simulink model "DemoMPEG"  (Simulink 7.7)
settings: Solver=ode45  StartTime=0.0  StopTime=10  RelTol=1e-3
PreLoadFcn:
  | EbNo = 16; Errors = 188; Bits = 1e8; M = 256; N = 64; Ts = (1/22050); constellation; InnerInterleaverBitTable
undefined symbols (not defined in the file or in its folder): gray, rsgenpoly
libraries: dspmtrx3 x33, simulink x18, commutil2 x6, commblkintrlv2 x4, commblkcod2 x2, vipsnks x2, dspindex x2, commseqgen2 x2, commrandsrc2 x2, commcnvintrlv2 x2, commsink2 x2, commcnvcod2 x2
settings Model: Creator=katsikas  LastModifiedBy=katsikas
settings SimEventsCC: propDiagAttribOutput=1  propDiagFcnCallOutput=1  propDiagStatOutput=0

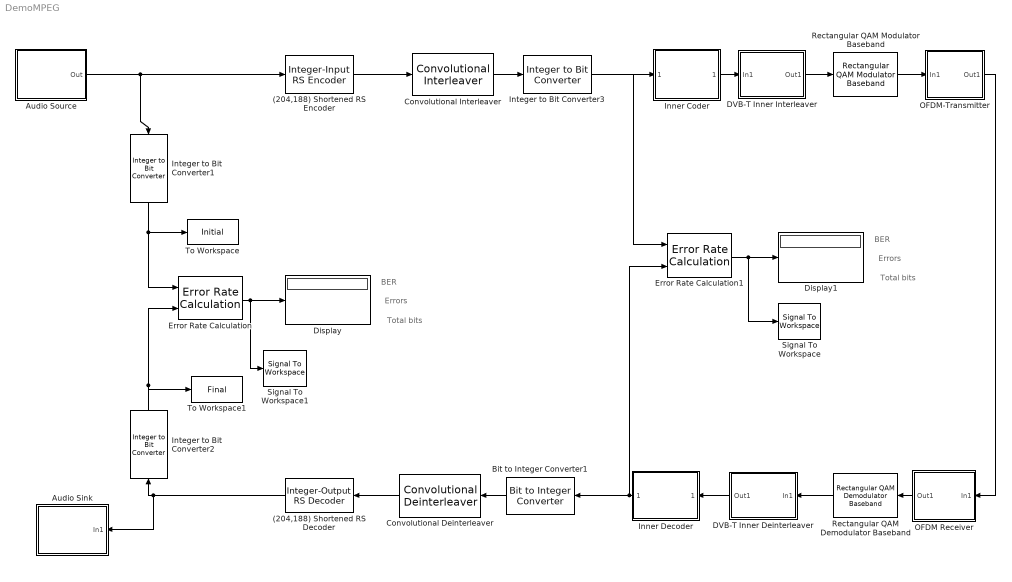
== system DemoMPEG ==
  note: BER
  note: Total bits
  note: Errors
  note: BER
  note: Total bits
  note: Errors
  (204,188) Shortened RS Decoder : commblkcod2/Integer-Output RS Decoder  n=204  k=188  specPrimPoly=off  prPoly=[1 0 1 1]  specGenPoly=off  genPoly=rsgenpoly(7,3)  specPuncture=off  punctVec=[ones(2,1); zeros(2,1)]  specErasurePort=off  showNumErr=off
  (204,188) Shortened RS Encoder : commblkcod2/Integer-Input RS Encoder  n=204  k=188  specPrimPoly=off  prPoly=[1 0 1 1]  specGenPoly=off  genPoly=rsgenpoly(7,3)  specPuncture=off  punctVec=[ones(2,1); zeros(2,1)]
  Audio Sink : Subsystem
  Audio Source : Subsystem
  Bit to Integer Converter1 : commutil2/Bit to Integer Converter  nbits=log2(M)  bitOrder=MSB first  signedOutputValues=Unsigned  outDtype=uint8  outDtypeSigned=Inherit via internal rule
  Convolutional Deinterleaver : commcnvintrlv2/Convolutional Deinterleaver  SystemSampleTime=-1  N=12  B=17  ic=0
  Convolutional Interleaver : commcnvintrlv2/Convolutional Interleaver  SystemSampleTime=-1  N=12  B=17  ic=0
  DVB-T Inner Deinterleaver : Subsystem  mask(DVB-T Inner Deinterleaver){}
      mask init:
      | fullILVec = [(1:126) ...
      |  (rem([0:125]+63,126) +1 + 126     ) ...
      |  (rem([0:125]+105,126)+1 + (2*126) ) ...
      |  (rem([0:125]+42,126) +1 + (3*126) ) ...
      |  (rem([0:125]+21,126) +1 + (4*126) ) ...
      |  (rem([0:125]+84,126) +1 + (5*126) )];
      mask Display: disp('DVB-T\nInner\nDeinterleaver')
  DVB-T Inner Interleaver : Subsystem  mask(DVB-T Inner Interleaver){}
      mask init: same as DemoMPEG/DVB-T Inner Deinterleaver
      mask Display: disp('DVB-T\nInner\nInterleaver')
  Display : Display
  Display1 : Display
  Error Rate Calculation : commsink2/Error Rate Calculation  N=188*17*8  st_delay=0  cp_mode=Entire frame  subframe=[]  PMode=Port  WsName=ErrorVec  RsMode2=off  stop=off  numErr=Errors  maxBits=Bits
  Error Rate Calculation1 : commsink2/Error Rate Calculation  N=1632*6  st_delay=0  cp_mode=Entire frame  subframe=[]  PMode=Port  WsName=ErrorVec  RsMode2=off  stop=off  numErr=100  maxBits=1e8
  Inner Coder : Subsystem
      mask Display: disp('Rate 3/4\nPunctured\nConvolutional\nCode');
  Inner Decoder : Subsystem
      mask Display: disp('Viterbi\nDecoder')
  Integer to Bit Converter1 : commutil2/Integer to Bit Converter  nbits=8  signedInputValues=Unsigned  bitOrder=MSB first  outDtype=boolean
  Integer to Bit Converter2 : commutil2/Integer to Bit Converter  nbits=8  signedInputValues=Unsigned  bitOrder=MSB first  outDtype=boolean
  Integer to Bit Converter3 : commutil2/Integer to Bit Converter  nbits=log2(M)  signedInputValues=Unsigned  bitOrder=MSB first  outDtype=boolean
  OFDM Receiver : Subsystem
  OFDM-Transmitter : Subsystem
  Rectangular QAM Demodulator Baseband : commdigbbndam3/Rectangular QAM Demodulator Baseband  M=N  PowType=Average Power  MinDist=2  AvgPow=1  PeakPow=1  Ph=0  Dec=User-defined  Mapping=map_constellation  OutType=Bit  DecType=Hard decision  VarSource=Dialog  Variance=1  outDtype1=boolean  outDtype2=Inherit via internal rule  derotateFactorWordLen=16  denormFactorWordLen=16  prodOutWordLen=32  prodOutRoundingMode=Floor  prodOutOverflowMode=Wrap  sumWordLen=32
  Rectangular QAM Modulator Baseband : commdigbbndam3/Rectangular QAM Modulator Baseband  M=N  InType=Bit  Enc=User-defined  Mapping=map_constellation  PowType=Average Power  MinDist=2  AvgPow=1  PeakPow=1  Ph=0  outDtype=double  outWordLen=16  outUDDataType=sfix(16)  outFracLenMode=Best precision  outFracLen=15
  Signal To Workspace : SignalToWorkspace  VariableName=BER1  SaveFormat=Array  Save2DMode=2-D array (concatenate along first dimension)
      settings: CopyFcn=dspblkcopystw(gcbh);
  Signal To Workspace1 : SignalToWorkspace  VariableName=BER  SaveFormat=Array  Save2DMode=2-D array (concatenate along first dimension)
      settings: CopyFcn=dspblkcopystw(gcbh);  MaxDataPoints=1
  To Workspace : ToWorkspace  VariableName=Initial  SampleTime=-1  SaveFormat=Array
  To Workspace1 : ToWorkspace  VariableName=Final  SampleTime=-1  SaveFormat=Array
  wires:
  Error Rate Calculation/1 -> Display/1, Signal To Workspace1/1
  Integer to Bit Converter2/1 -> Error Rate Calculation/2, To Workspace1/1
  (204,188) Shortened RS Decoder/1 -> Integer to Bit Converter2/1, Audio Sink/1(In1)
  Rectangular QAM Modulator Baseband/1 -> OFDM-Transmitter/1(In1)
  Convolutional Interleaver/1 -> Integer to Bit Converter3/1
  Convolutional Deinterleaver/1 -> (204,188) Shortened RS Decoder/1
  (204,188) Shortened RS Encoder/1 -> Convolutional Interleaver/1
  Error Rate Calculation1/1 -> Display1/1, Signal To Workspace/1
  Integer to Bit Converter3/1 -> Inner Coder/1(Uncoded symbols), Error Rate Calculation1/1
  Rectangular QAM Demodulator Baseband/1 -> DVB-T Inner Deinterleaver/1(In1)
  Bit to Integer Converter1/1 -> Convolutional Deinterleaver/1
  Inner Coder/1(Coded bits) -> DVB-T Inner Interleaver/1(In1)
  Inner Decoder/1(Decoded symbols) -> Bit to Integer Converter1/1, Error Rate Calculation1/2
  DVB-T Inner Interleaver/1(Out1) -> Rectangular QAM Modulator Baseband/1
  DVB-T Inner Deinterleaver/1(Out1) -> Inner Decoder/1(Received bits)
  OFDM Receiver/1(Out1) -> Rectangular QAM Demodulator Baseband/1
  OFDM-Transmitter/1(Out1) -> OFDM Receiver/1(In1)
  Integer to Bit Converter1/1 -> Error Rate Calculation/1, To Workspace/1
  Audio Source/1(Out) -> Integer to Bit Converter1/1, (204,188) Shortened RS Encoder/1

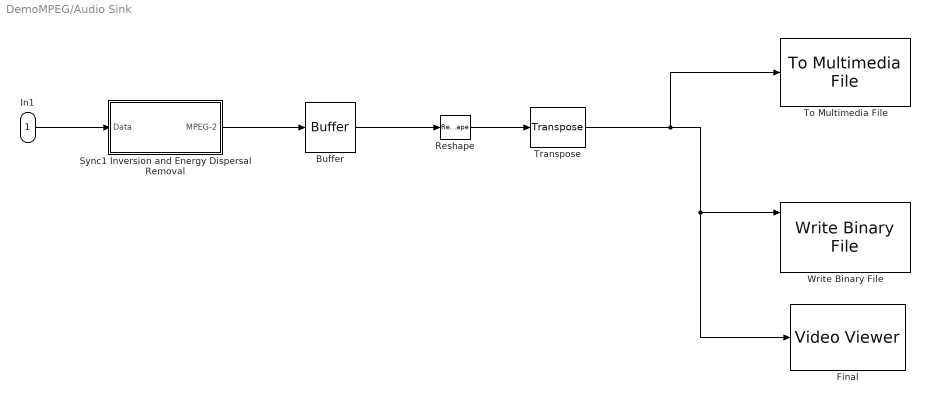
== system DemoMPEG/Audio Sink ==
  In1 : Inport
  Buffer : Buffer  N=120*160  TreatMby1Signals=One channel
  Final : vipsnks/Video Viewer  inputType=Obsolete7b  imagePorts=One multidimensional signal  useColorMap=off  colormapValue=gray(256)  specRange=off  minInputVal=0  maxInputVal=255  FigPos=[730 1122 458 411]  AxisZoom=on  trueSizedOnce=on  OpenAtMdlStart=on
  Reshape : Reshape  OutputDimensionality=Customize  OutputDimensions=[160,120]
  Sync1 Inversion and Energy Dispersal Removal : Subsystem
  To Multimedia File : dspsnks4/To Multimedia File  outputFilename=output.avi  streamSelection=Video only  videoCompressor=None (uncompressed)  audioCompressor=None (uncompressed)  imagePorts=One multidimensional signal  fileType=AVI  audioDatatype=Determine from input data type  fourcc=RGB
  Transpose : dspmtrx3/Transpose  SystemSampleTime=-1  Hermitian=off  overflowFlag=off
  Write Binary File : vipsnks/Write Binary File  FileName=output.bin  VideoFormat=Four character codes  FOURCC=I420  BitStreamFormat=Planar  NumInputs=3  ComponentOrder=[1 2 3]  Interlaced=off  LineOrdering=Top line first  InheritBits=on  Component1=Y'  Component2=Cb  Component3=Cr  Component4=Alpha  Bits1=8  Bits2=8  Bits3=8  Bits4=0  SignedInput=off  FileEndian=Little endian
  wires:
  Reshape/1 -> Transpose/1
  Buffer/1 -> Reshape/1
  In1/1 -> Sync1 Inversion and Energy Dispersal Removal/1(Data)
  Transpose/1 -> Final/1, Write Binary File/1, To Multimedia File/1
  Sync1 Inversion and Energy Dispersal Removal/1(MPEG-2) -> Buffer/1

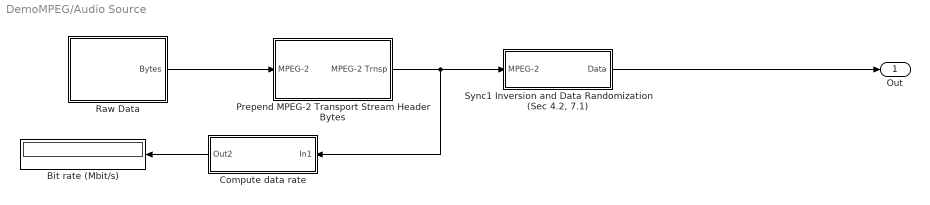
== system DemoMPEG/Audio Source ==
  Bit rate (Mbit/s) : Display
      settings: Format=bank
  Compute data rate : Subsystem
      mask Display: disp(sprintf('Compute Bit\nRate (Mbit/s)'))
  Prepend MPEG-2 Transport Stream Header Bytes : Subsystem
      mask Display: disp(sprintf('Prepend MPEG-2\nTransportStream\nHeader Bytes'))
  "Raw Data " : Subsystem
  "Sync1 Inversion and Data Randomization (Sec 4.2, 7.1)" : Subsystem
  Out : Outport
  wires:
  Prepend MPEG-2 Transport Stream Header Bytes/1(MPEG-2 Trnsp) -> "Sync1 Inversion and Data Randomization (Sec 4.2, 7.1)"/1(MPEG-2), Compute data rate/1(In1)
  "Sync1 Inversion and Data Randomization (Sec 4.2, 7.1)"/1(Data) -> Out/1
  "Raw Data "/1(Bytes) -> Prepend MPEG-2 Transport Stream Header Bytes/1(MPEG-2)
  Compute data rate/1(Out2) -> Bit rate (Mbit/s)/1

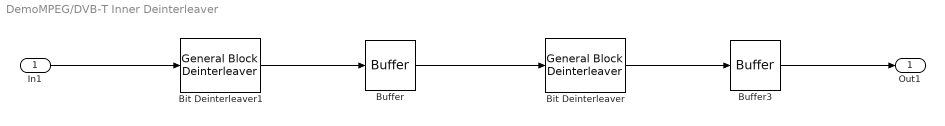
== system DemoMPEG/DVB-T Inner Deinterleaver ==
  In1 : Inport
  Bit Deinterleaver : commblkintrlv2/General Block Deinterleaver  elements=BitInterleaverTable
  Bit Deinterleaver1 : commblkintrlv2/General Block Deinterleaver  elements=SymbolInterleaverTable
  Buffer : Buffer  N=756  TreatMby1Signals=One channel
  Buffer3 : Buffer  N=2176  TreatMby1Signals=One channel
  Out1 : Outport
  wires:
  In1/1 -> Bit Deinterleaver1/1
  Buffer3/1 -> Out1/1
  Buffer/1 -> Bit Deinterleaver/1
  Bit Deinterleaver/1 -> Buffer3/1
  Bit Deinterleaver1/1 -> Buffer/1

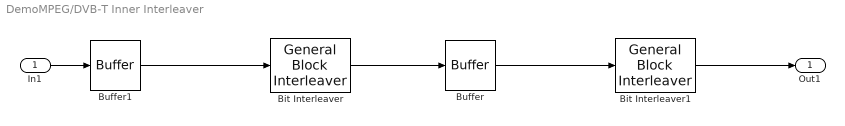
== system DemoMPEG/DVB-T Inner Interleaver ==
  In1 : Inport
  Bit Interleaver : commblkintrlv2/General Block Interleaver  elements=BitInterleaverTable
  Bit Interleaver1 : commblkintrlv2/General Block Interleaver  elements=SymbolInterleaverTable
  Buffer : Buffer  N=9072  TreatMby1Signals=One channel
  Buffer1 : Buffer  N=756  TreatMby1Signals=One channel
  Out1 : Outport
  wires:
  In1/1 -> Buffer1/1
  Buffer/1 -> Bit Interleaver1/1
  Buffer1/1 -> Bit Interleaver/1
  Bit Interleaver/1 -> Buffer/1
  Bit Interleaver1/1 -> Out1/1

== system DemoMPEG/Inner Coder ==
  Uncoded symbols : Inport
  Convolutional  Encoder : commcnvcod2/Convolutional Encoder  trellis=poly2trellis(7, [171 133])  opMode=Continuous  DelayedResetAction=off  hasIniStPort=off  hasFinStPort=off  usePuncVector=on  punctureVector=[1 1 0 1 1 0]'  reset=Unused parameter value
  Coded bits : Outport
  wires:
  Convolutional  Encoder/1 -> Coded bits/1
  Uncoded symbols/1 -> Convolutional  Encoder/1

== system DemoMPEG/Inner Decoder ==
  note: Align on 1632-bit
      | frame boundary
  Received bits : Inport
  Delay : dspsigops/Delay  InputProcessing=Columns as channels (frame based)  dly_unit=Samples  delay=584+69  ic_detail=off  dif_ic_for_ch=off  dif_ic_for_dly=off  ic=0  reset_popup=None
  Viterbi Decoder : commcnvcod2/Viterbi Decoder  trellis=poly2trellis(7, [171 133])  isPunctured=on  punctureVector=[1 1 0 1 1 0]'  erasures=off  dectype=Hard decision  runSigValErrCheck=off  nsdecb=4  smWordLength=16  tbdepth=136  opmode=Continuous  reset=off  outDataType=boolean
  Decoded symbols : Outport
  wires:
  Viterbi Decoder/1 -> Delay/1
  Received bits/1 -> Viterbi Decoder/1
  Delay/1 -> Decoded symbols/1

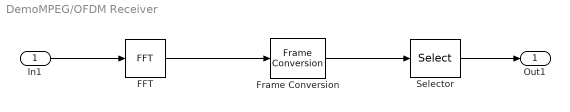
== system DemoMPEG/OFDM Receiver ==
  In1 : Inport
  FFT : dspxfrm3/FFT  CompMethod=Table lookup  TableOpt=NEW  TableOptActive=Speed  BitRevOrder=off  InheritFFTLength=on  FFTLength=64  RowConvenienceOn=on  SkipNorm=off  firstCoeffDataTypeStr=Inherit: Same word length as input  firstCoeffLastDataTypeStr=Inherit: Same word length as input  outputMin=[]  outputMax=[]  roundingMode=Floor  overflowMode=off
  Frame Conversion : FrameConversion
  Selector : Selector  NumberOfDimensions=2  InputPortWidth=3  IndexOptions=Index vector (dialog),Select all  Indices=[1:756 1293:2048],1  OutputSizes=1,1
  Out1 : Outport
  wires:
  FFT/1 -> Frame Conversion/1
  Frame Conversion/1 -> Selector/1
  In1/1 -> FFT/1
  Selector/1 -> Out1/1

== system DemoMPEG/OFDM-Transmitter ==
  In1 : Inport
  IFFT : dspxfrm3/IFFT  CompMethod=Table lookup  TableOpt=NEW  TableOptActive=Speed  BitRevOrder=off  cs_in=off  SkipNorm=on  InheritFFTLength=on  FFTLength=64  mode=Complex  outSamplingMode=Frame based  RowConvenienceOn=on  firstCoeffDataTypeStr=Inherit: Same word length as input  firstCoeffLastDataTypeStr=Inherit: Same word length as input  outputMin=[]  outputMax=[]  roundingMode=Floor  overflowMode=off
  Pad : dspsigops/Pad  padAlong=Columns  dimsToPad=1  valSrc=Specify via dialog  padVal=0  spec=Output size  padNumOutRowsSpecMethod=User-specified  numOutRows=2048  padNumOutColsSpecMethod=User-specified  numOutCols=1  isVarDimsMode=off  padBeginning=0  padEnd=0  outSizeMode=User-specified  outSize=1  padSigAt=End  trunc_flag=None  roundingMode=Floor  overflowMode=off  truncOrWrapMode=Truncate  wrap_flag=None
  Selector : Selector  NumberOfDimensions=2  InputPortWidth=3  IndexOptions=Index vector (dialog),Select all  Indices=[1:756 1513:2048 757:1512],1  OutputSizes=1,1
  Out1 : Outport
  wires:
  Pad/1 -> Selector/1
  Selector/1 -> IFFT/1
  IFFT/1 -> Out1/1
  In1/1 -> Pad/1

== system DemoMPEG/Audio Sink/Sync1 Inversion and Energy Dispersal Removal ==
  Data : Inport
  Buffer to Superframes : Buffer  N=1504  TreatMby1Signals=One channel
  Rebuffer to Packets : Buffer  N=188  TreatMby1Signals=One channel
  Scrambler-Descrambler : Subsystem
  MPEG-2 : Outport
  wires:
  Data/1 -> Buffer to Superframes/1
  Rebuffer to Packets/1 -> MPEG-2/1
  Buffer to Superframes/1 -> Scrambler-Descrambler/1(Data_In)
  Scrambler-Descrambler/1(Data_Out) -> Rebuffer to Packets/1

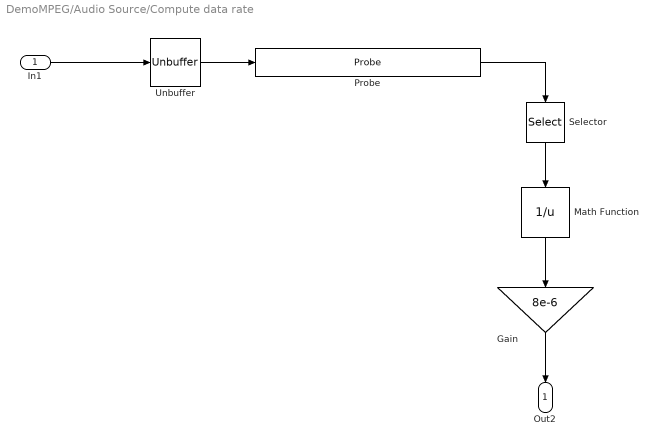
== system DemoMPEG/Audio Source/Compute data rate ==
  In1 : Inport
  Gain : Gain  Gain=8e-6
  Math Function : Math  Operator=reciprocal  SaturateOnIntegerOverflow=on
  Probe : Probe  ProbeWidth=off  ProbeComplexSignal=off
  Selector : Selector  InputPortWidth=2  IndexOptions=Index vector (dialog)  Indices=1  OutputSizes=1
  Unbuffer : Unbuffer  SampleBasedProcessing=Same as frame based
  Out2 : Outport
  wires:
  Probe/1 -> Selector/1
  In1/1 -> Unbuffer/1
  Selector/1 -> Math Function/1
  Math Function/1 -> Gain/1
  Gain/1 -> Out2/1
  Unbuffer/1 -> Probe/1

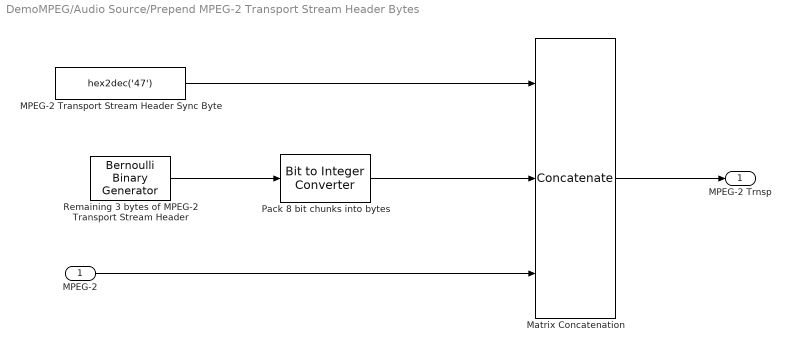
== system DemoMPEG/Audio Source/Prepend MPEG-2 Transport Stream Header Bytes ==
  MPEG-2 : Inport
  MPEG-2 Transport Stream Header Sync Byte : Constant  Value=hex2dec('47')  VectorParams1D=off  OutDataTypeStr=uint8  FramePeriod=(8*188)/9.6e6
      settings: SamplingMode=Frame based
  Matrix Concatenation : Concatenate  NumInputs=3  Mode=Multidimensional array
  Pack 8 bit chunks into bytes : commutil2/Bit to Integer Converter  nbits=8  bitOrder=MSB first  signedOutputValues=Unsigned  outDtype=uint8  outDtypeSigned=Inherit via internal rule
  Remaining 3 bytes of MPEG-2 Transport Stream Header : commrandsrc2/Bernoulli Binary Generator  SystemSampleTime=-1  P=0.5  seed=61  Ts=(8*188/9.6e6) / (3*8)  frameBased=on  sampPerFrame=3*8  orient=off  outDataType=uint8
  MPEG-2 Trnsp : Outport
  wires:
  MPEG-2 Transport Stream Header Sync Byte/1 -> Matrix Concatenation/1
  Remaining 3 bytes of MPEG-2 Transport Stream Header/1 -> Pack 8 bit chunks into bytes/1
  Matrix Concatenation/1 -> MPEG-2 Trnsp/1
  Pack 8 bit chunks into bytes/1 -> Matrix Concatenation/2
  MPEG-2/1 -> Matrix Concatenation/3

== system DemoMPEG/Audio Source/Raw Data  ==
  184 bytes of MPEG-2 or auxiliary data : commrandsrc2/Bernoulli Binary Generator  SystemSampleTime=-1  P=0.5  seed=61  Ts=(8*188/9.6e6) / (8 * 184)  frameBased=on  sampPerFrame=8 * 184  orient=off  outDataType=uint8
  Pack 8 bit chunks into bytes : commutil2/Bit to Integer Converter  nbits=8  bitOrder=MSB first  signedOutputValues=Unsigned  outDtype=uint8  outDtypeSigned=Inherit via internal rule
  Bytes : Outport
  wires:
  184 bytes of MPEG-2 or auxiliary data/1 -> Pack 8 bit chunks into bytes/1
  Pack 8 bit chunks into bytes/1 -> Bytes/1

== system DemoMPEG/Audio Source/Sync1 Inversion and Data Randomization (Sec 4.2, 7.1) ==
  MPEG-2 : Inport
  Buffer to Superframes : Buffer  N=1504  TreatMby1Signals=One channel
  Rebuffer to Packets : Buffer  N=188  TreatMby1Signals=One channel
  Scrambler-Descrambler : Subsystem
  Data : Outport
  wires:
  MPEG-2/1 -> Buffer to Superframes/1
  Rebuffer to Packets/1 -> Data/1
  Scrambler-Descrambler/1(Data_Out) -> Rebuffer to Packets/1
  Buffer to Superframes/1 -> Scrambler-Descrambler/1(Data_In)

== system DemoMPEG/Audio Sink/Sync1 Inversion and Energy Dispersal Removal/Scrambler-Descrambler ==
  Data_In : Inport
  PRBS : Subsystem
  XOR and Concatenate : Subsystem
  Data_Out : Outport
  wires:
  PRBS/1(PRBS1) -> XOR and Concatenate/2(PRBS1)
  PRBS/2(PRBS2) -> XOR and Concatenate/3(PRBS2)
  PRBS/3(PRBS3) -> XOR and Concatenate/4(PRBS3)
  PRBS/4(PRBS4) -> XOR and Concatenate/5(PRBS4)
  PRBS/5(PRBS5) -> XOR and Concatenate/6(PRBS5)
  PRBS/6(PRBS6) -> XOR and Concatenate/7(PRBS6)
  PRBS/7(PRBS7) -> XOR and Concatenate/8(PRBS7)
  PRBS/8(PRBS8) -> XOR and Concatenate/9(PRBS8)
  Data_In/1 -> XOR and Concatenate/1(Data)
  XOR and Concatenate/1(Out1) -> Data_Out/1

== system DemoMPEG/Audio Source/Sync1 Inversion and Data Randomization (Sec 4.2, 7.1)/Scrambler-Descrambler ==
  Data_In : Inport
  PRBS : Subsystem
  XOR and Concatenate : Subsystem
  Data_Out : Outport
  wires:
  PRBS/1(PRBS1) -> XOR and Concatenate/2(PRBS1)
  PRBS/2(PRBS2) -> XOR and Concatenate/3(PRBS2)
  PRBS/3(PRBS3) -> XOR and Concatenate/4(PRBS3)
  PRBS/4(PRBS4) -> XOR and Concatenate/5(PRBS4)
  PRBS/5(PRBS5) -> XOR and Concatenate/6(PRBS5)
  PRBS/6(PRBS6) -> XOR and Concatenate/7(PRBS6)
  PRBS/7(PRBS7) -> XOR and Concatenate/8(PRBS7)
  PRBS/8(PRBS8) -> XOR and Concatenate/9(PRBS8)
  Data_In/1 -> XOR and Concatenate/1(Data)
  XOR and Concatenate/1(Out1) -> Data_Out/1

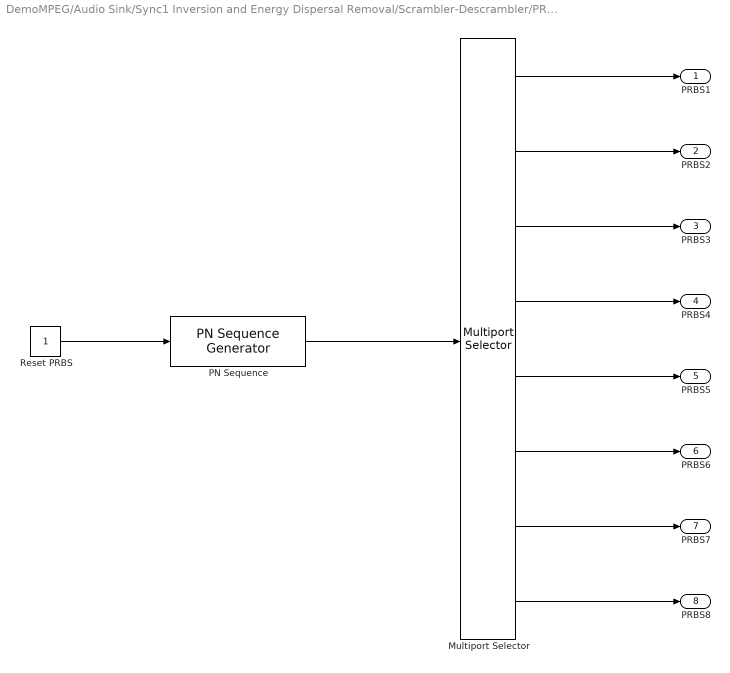
== system DemoMPEG/Audio Sink/Sync1 Inversion and Energy Dispersal Removal/Scrambler-Descrambler/PRBS ==
  Multiport Selector : dspindex/Multiport Selector  rowsOrCols=Rows  idxCellArray={[1:187], [189:375], [377:563], [565:751], [753:939], [941:1127], [1129:1315], [1317:1503]}  idxErrMode=Clip Index
  PN Sequence : commseqgen2/PN Sequence Generator  poly=[15 1 0]  ini_sta=[1 0 0 1 0 1 0 1 0 0 0 0 0 0 0]  outBitMaskSource=Dialog parameter  shift=15  outVarSiz=off  maxOutSizeMode=Dialog parameter  maxOutSize=[10 1]  Ts=8 * (8*188/9.6e6) / (8*188 - 1)  frameBased=on  sampPerFrame=(8*188 - 1)  reset=on  bitPackedOutputs=on  outDataType=Smallest unsigned integer  numPackedBits=8  bitPackDataSigned=off  bitPackedOutDType=Smallest integer
  Reset PRBS : Constant  VectorParams1D=off  OutDataTypeStr=boolean  SampleTime=8 * (8*188/9.6e6)
  PRBS1 : Outport
  PRBS2 : Outport  Port=2
  PRBS3 : Outport  Port=3
  PRBS4 : Outport  Port=4
  PRBS5 : Outport  Port=5
  PRBS6 : Outport  Port=6
  PRBS7 : Outport  Port=7
  PRBS8 : Outport  Port=8
  wires:
  PN Sequence/1 -> Multiport Selector/1
  Multiport Selector/1 -> PRBS1/1
  Multiport Selector/2 -> PRBS2/1
  Multiport Selector/3 -> PRBS3/1
  Multiport Selector/4 -> PRBS4/1
  Multiport Selector/5 -> PRBS5/1
  Multiport Selector/6 -> PRBS6/1
  Multiport Selector/7 -> PRBS7/1
  Multiport Selector/8 -> PRBS8/1
  Reset PRBS/1 -> PN Sequence/1

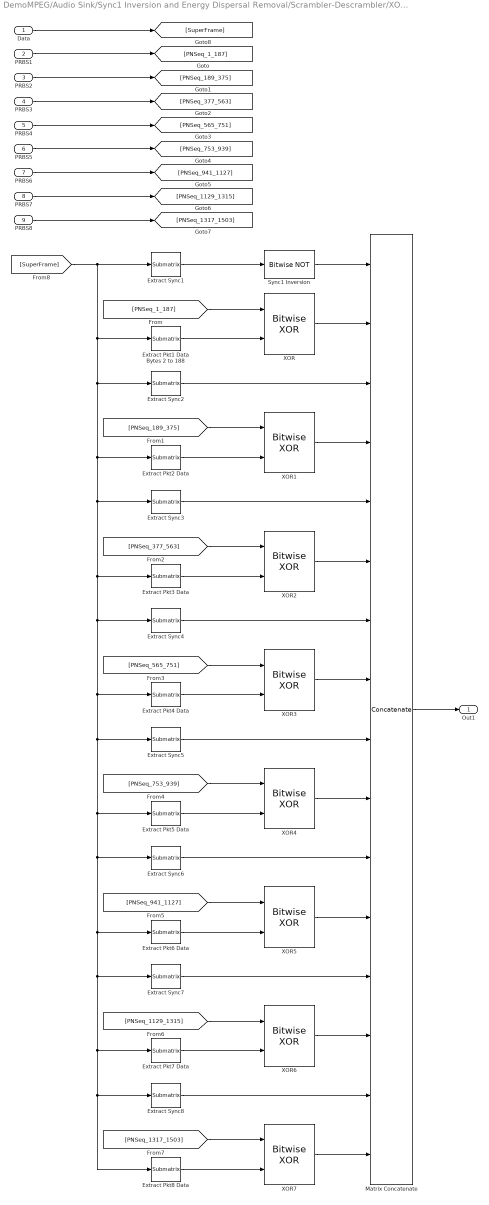
== system DemoMPEG/Audio Sink/Sync1 Inversion and Energy Dispersal Removal/Scrambler-Descrambler/XOR and Concatenate ==
  Data : Inport
  PRBS1 : Inport  Port=2
  PRBS2 : Inport  Port=3
  PRBS3 : Inport  Port=4
  PRBS4 : Inport  Port=5
  PRBS5 : Inport  Port=6
  PRBS6 : Inport  Port=7
  PRBS7 : Inport  Port=8
  PRBS8 : Inport  Port=9
  Extract Pkt1 Data Bytes 2 to 188 : dspmtrx3/Submatrix  RowSpan=Range of rows  RowStartMode=Index  RowStartIndex=2  RowEndMode=Index  RowEndIndex=188  ColSpan=All columns  ColStartMode=First  ColStartIndex=1  ColEndMode=Last  ColEndIndex=1
  Extract Pkt2 Data : dspmtrx3/Submatrix  RowSpan=Range of rows  RowStartMode=Index  RowStartIndex=188+2  RowEndMode=Index  RowEndIndex=2*188  ColSpan=All columns  ColStartMode=First  ColStartIndex=1  ColEndMode=Last  ColEndIndex=1
  Extract Pkt3 Data : dspmtrx3/Submatrix  RowSpan=Range of rows  RowStartMode=Index  RowStartIndex=2*188+2  RowEndMode=Index  RowEndIndex=3*188  ColSpan=All columns  ColStartMode=First  ColStartIndex=1  ColEndMode=Last  ColEndIndex=1
  Extract Pkt4 Data : dspmtrx3/Submatrix  RowSpan=Range of rows  RowStartMode=Index  RowStartIndex=3*188+2  RowEndMode=Index  RowEndIndex=4*188  ColSpan=All columns  ColStartMode=First  ColStartIndex=1  ColEndMode=Last  ColEndIndex=1
  Extract Pkt5 Data : dspmtrx3/Submatrix  RowSpan=Range of rows  RowStartMode=Index  RowStartIndex=4*188+2  RowEndMode=Index  RowEndIndex=5*188  ColSpan=All columns  ColStartMode=First  ColStartIndex=1  ColEndMode=Last  ColEndIndex=1
  Extract Pkt6 Data : dspmtrx3/Submatrix  RowSpan=Range of rows  RowStartMode=Index  RowStartIndex=5*188+2  RowEndMode=Index  RowEndIndex=6*188  ColSpan=All columns  ColStartMode=First  ColStartIndex=1  ColEndMode=Last  ColEndIndex=1
  Extract Pkt7 Data : dspmtrx3/Submatrix  RowSpan=Range of rows  RowStartMode=Index  RowStartIndex=6*188+2  RowEndMode=Index  RowEndIndex=7*188  ColSpan=All columns  ColStartMode=First  ColStartIndex=1  ColEndMode=Last  ColEndIndex=1
  Extract Pkt8 Data : dspmtrx3/Submatrix  RowSpan=Range of rows  RowStartMode=Index  RowStartIndex=7*188+2  RowEndMode=Last  RowEndIndex=8*188  ColSpan=All columns  ColStartMode=First  ColStartIndex=1  ColEndMode=Last  ColEndIndex=1
  Extract Sync1 : dspmtrx3/Submatrix  RowSpan=One row  RowStartMode=First  RowStartIndex=1  RowEndMode=Index  RowEndIndex=8  ColSpan=All columns  ColStartMode=First  ColStartIndex=1  ColEndMode=Last  ColEndIndex=1
  Extract Sync2 : dspmtrx3/Submatrix  RowSpan=One row  RowStartMode=Index  RowStartIndex=188+1  RowEndMode=Index  RowEndIndex=8  ColSpan=All columns  ColStartMode=First  ColStartIndex=1  ColEndMode=Last  ColEndIndex=1
  Extract Sync3 : dspmtrx3/Submatrix  RowSpan=One row  RowStartMode=Index  RowStartIndex=2*188+1  RowEndMode=Index  RowEndIndex=8  ColSpan=All columns  ColStartMode=First  ColStartIndex=1  ColEndMode=Last  ColEndIndex=1
  Extract Sync4 : dspmtrx3/Submatrix  RowSpan=One row  RowStartMode=Index  RowStartIndex=3*188+1  RowEndMode=Index  RowEndIndex=8  ColSpan=All columns  ColStartMode=First  ColStartIndex=1  ColEndMode=Last  ColEndIndex=1
  Extract Sync5 : dspmtrx3/Submatrix  RowSpan=One row  RowStartMode=Index  RowStartIndex=4*188+1  RowEndMode=Index  RowEndIndex=8  ColSpan=All columns  ColStartMode=First  ColStartIndex=1  ColEndMode=Last  ColEndIndex=1
  Extract Sync6 : dspmtrx3/Submatrix  RowSpan=One row  RowStartMode=Index  RowStartIndex=5*188+1  RowEndMode=Index  RowEndIndex=8  ColSpan=All columns  ColStartMode=First  ColStartIndex=1  ColEndMode=Last  ColEndIndex=1
  Extract Sync7 : dspmtrx3/Submatrix  RowSpan=One row  RowStartMode=Index  RowStartIndex=6*188+1  RowEndMode=Index  RowEndIndex=8  ColSpan=All columns  ColStartMode=First  ColStartIndex=1  ColEndMode=Last  ColEndIndex=1
  Extract Sync8 : dspmtrx3/Submatrix  RowSpan=One row  RowStartMode=Index  RowStartIndex=7*188+1  RowEndMode=Index  RowEndIndex=8  ColSpan=All columns  ColStartMode=First  ColStartIndex=1  ColEndMode=Last  ColEndIndex=1
  Matrix Concatenate : Concatenate  NumInputs=16  Mode=Multidimensional array
  Sync1 Inversion : simulink/Logic and Bit Operations/Bitwise Operator  logicop=NOT  UseBitMask=off  BitMask=bin2dec('11011001')  BitMaskRealWorld=Stored Integer
  XOR{,1..7} (8 alike) : simulink/Logic and Bit Operations/Bitwise Operator  logicop=XOR  UseBitMask=off  NumInputPorts=2  BitMask=bin2dec('11011001')  BitMaskRealWorld=Stored Integer
  Out1 : Outport
  wires:
  [SuperFrame] -> Extract Pkt2 Data/1, Extract Pkt3 Data/1, Extract Pkt4 Data/1, Extract Pkt5 Data/1, Extract Pkt6 Data/1, Extract Pkt8 Data/1, Extract Sync8/1, Extract Pkt7 Data/1, Extract Sync7/1, Extract Sync6/1, Extract Sync5/1, Extract Sync4/1, Extract Sync3/1, Extract Sync2/1, Extract Pkt1 Data Bytes 2 to 188/1, Extract Sync1/1
  Extract Sync1/1 -> Sync1 Inversion/1
  Extract Pkt1 Data Bytes 2 to 188/1 -> XOR/2
  [PNSeq_1_187] -> XOR/1
  Sync1 Inversion/1 -> Matrix Concatenate/1
  XOR/1 -> Matrix Concatenate/2
  Extract Sync2/1 -> Matrix Concatenate/3
  Extract Sync3/1 -> Matrix Concatenate/5
  Extract Sync4/1 -> Matrix Concatenate/7
  Extract Sync5/1 -> Matrix Concatenate/9
  Extract Sync6/1 -> Matrix Concatenate/11
  Extract Sync7/1 -> Matrix Concatenate/13
  Extract Sync8/1 -> Matrix Concatenate/15
  XOR1/1 -> Matrix Concatenate/4
  XOR2/1 -> Matrix Concatenate/6
  XOR3/1 -> Matrix Concatenate/8
  XOR4/1 -> Matrix Concatenate/10
  XOR5/1 -> Matrix Concatenate/12
  XOR6/1 -> Matrix Concatenate/14
  XOR7/1 -> Matrix Concatenate/16
  [PNSeq_189_375] -> XOR1/1
  [PNSeq_377_563] -> XOR2/1
  [PNSeq_565_751] -> XOR3/1
  [PNSeq_753_939] -> XOR4/1
  [PNSeq_941_1127] -> XOR5/1
  [PNSeq_1129_1315] -> XOR6/1
  [PNSeq_1317_1503] -> XOR7/1
  Extract Pkt2 Data/1 -> XOR1/2
  Extract Pkt3 Data/1 -> XOR2/2
  Extract Pkt4 Data/1 -> XOR3/2
  Extract Pkt5 Data/1 -> XOR4/2
  Extract Pkt6 Data/1 -> XOR5/2
  Extract Pkt7 Data/1 -> XOR6/2
  Extract Pkt8 Data/1 -> XOR7/2
  Matrix Concatenate/1 -> Out1/1
  PRBS1/1 -> [PNSeq_1_187]
  PRBS2/1 -> [PNSeq_189_375]
  PRBS3/1 -> [PNSeq_377_563]
  PRBS4/1 -> [PNSeq_565_751]
  PRBS5/1 -> [PNSeq_753_939]
  PRBS6/1 -> [PNSeq_941_1127]
  PRBS7/1 -> [PNSeq_1129_1315]
  PRBS8/1 -> [PNSeq_1317_1503]
  Data/1 -> [SuperFrame]

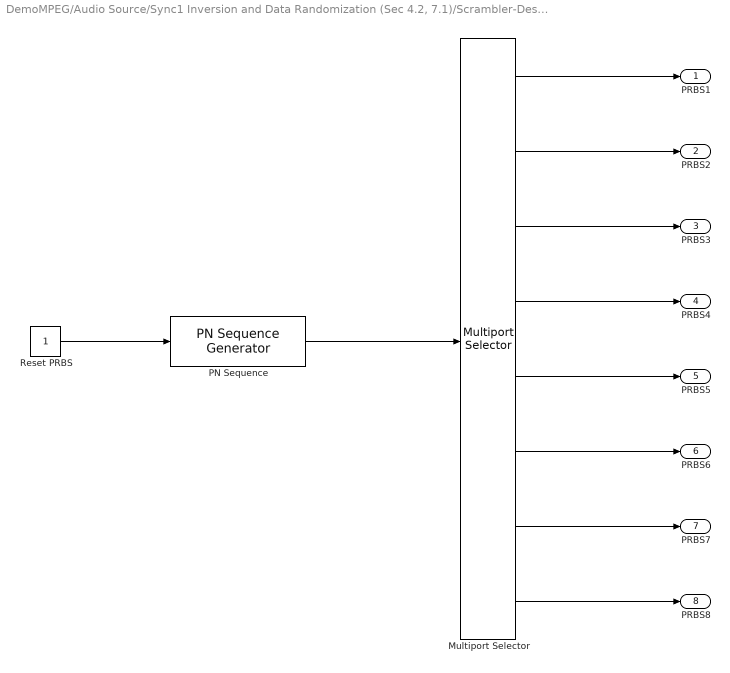
== system DemoMPEG/Audio Source/Sync1 Inversion and Data Randomization (Sec 4.2, 7.1)/Scrambler-Descrambler/PRBS ==
  Multiport Selector : dspindex/Multiport Selector  rowsOrCols=Rows  idxCellArray={[1:187], [189:375], [377:563], [565:751], [753:939], [941:1127], [1129:1315], [1317:1503]}  idxErrMode=Clip Index
  PN Sequence : commseqgen2/PN Sequence Generator  poly=[15 1 0]  ini_sta=[1 0 0 1 0 1 0 1 0 0 0 0 0 0 0]  outBitMaskSource=Dialog parameter  shift=15  outVarSiz=off  maxOutSizeMode=Dialog parameter  maxOutSize=[10 1]  Ts=8 * (8*188/9.6e6) / (8*188 - 1)  frameBased=on  sampPerFrame=(8*188 - 1)  reset=on  bitPackedOutputs=on  outDataType=Smallest unsigned integer  numPackedBits=8  bitPackDataSigned=off  bitPackedOutDType=Smallest integer
  Reset PRBS : Constant  VectorParams1D=off  OutDataTypeStr=boolean  SampleTime=8 * (8*188/9.6e6)
  PRBS1 : Outport
  PRBS2 : Outport  Port=2
  PRBS3 : Outport  Port=3
  PRBS4 : Outport  Port=4
  PRBS5 : Outport  Port=5
  PRBS6 : Outport  Port=6
  PRBS7 : Outport  Port=7
  PRBS8 : Outport  Port=8
  wires:
  Multiport Selector/1 -> PRBS1/1
  Multiport Selector/2 -> PRBS2/1
  Multiport Selector/3 -> PRBS3/1
  Multiport Selector/4 -> PRBS4/1
  Multiport Selector/5 -> PRBS5/1
  Multiport Selector/6 -> PRBS6/1
  Multiport Selector/7 -> PRBS7/1
  Multiport Selector/8 -> PRBS8/1
  PN Sequence/1 -> Multiport Selector/1
  Reset PRBS/1 -> PN Sequence/1

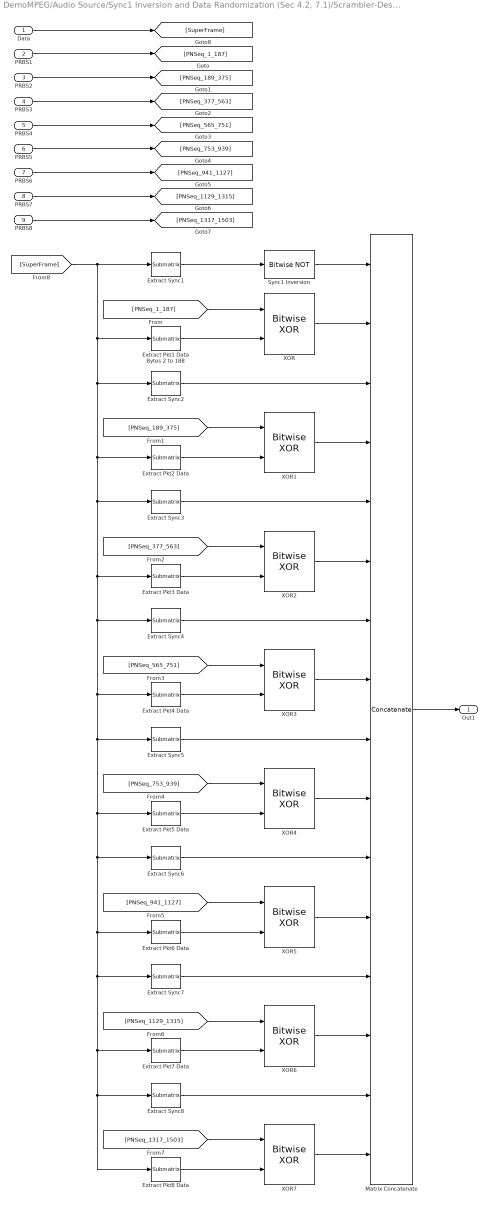
== system DemoMPEG/Audio Source/Sync1 Inversion and Data Randomization (Sec 4.2, 7.1)/Scrambler-Descrambler/XOR and Concatenate ==
  Data : Inport
  PRBS1 : Inport  Port=2
  PRBS2 : Inport  Port=3
  PRBS3 : Inport  Port=4
  PRBS4 : Inport  Port=5
  PRBS5 : Inport  Port=6
  PRBS6 : Inport  Port=7
  PRBS7 : Inport  Port=8
  PRBS8 : Inport  Port=9
  Extract Pkt1 Data Bytes 2 to 188 : dspmtrx3/Submatrix  RowSpan=Range of rows  RowStartMode=Index  RowStartIndex=2  RowEndMode=Index  RowEndIndex=188  ColSpan=All columns  ColStartMode=First  ColStartIndex=1  ColEndMode=Last  ColEndIndex=1
  Extract Pkt2 Data : dspmtrx3/Submatrix  RowSpan=Range of rows  RowStartMode=Index  RowStartIndex=188+2  RowEndMode=Index  RowEndIndex=2*188  ColSpan=All columns  ColStartMode=First  ColStartIndex=1  ColEndMode=Last  ColEndIndex=1
  Extract Pkt3 Data : dspmtrx3/Submatrix  RowSpan=Range of rows  RowStartMode=Index  RowStartIndex=2*188+2  RowEndMode=Index  RowEndIndex=3*188  ColSpan=All columns  ColStartMode=First  ColStartIndex=1  ColEndMode=Last  ColEndIndex=1
  Extract Pkt4 Data : dspmtrx3/Submatrix  RowSpan=Range of rows  RowStartMode=Index  RowStartIndex=3*188+2  RowEndMode=Index  RowEndIndex=4*188  ColSpan=All columns  ColStartMode=First  ColStartIndex=1  ColEndMode=Last  ColEndIndex=1
  Extract Pkt5 Data : dspmtrx3/Submatrix  RowSpan=Range of rows  RowStartMode=Index  RowStartIndex=4*188+2  RowEndMode=Index  RowEndIndex=5*188  ColSpan=All columns  ColStartMode=First  ColStartIndex=1  ColEndMode=Last  ColEndIndex=1
  Extract Pkt6 Data : dspmtrx3/Submatrix  RowSpan=Range of rows  RowStartMode=Index  RowStartIndex=5*188+2  RowEndMode=Index  RowEndIndex=6*188  ColSpan=All columns  ColStartMode=First  ColStartIndex=1  ColEndMode=Last  ColEndIndex=1
  Extract Pkt7 Data : dspmtrx3/Submatrix  RowSpan=Range of rows  RowStartMode=Index  RowStartIndex=6*188+2  RowEndMode=Index  RowEndIndex=7*188  ColSpan=All columns  ColStartMode=First  ColStartIndex=1  ColEndMode=Last  ColEndIndex=1
  Extract Pkt8 Data : dspmtrx3/Submatrix  RowSpan=Range of rows  RowStartMode=Index  RowStartIndex=7*188+2  RowEndMode=Last  RowEndIndex=8*188  ColSpan=All columns  ColStartMode=First  ColStartIndex=1  ColEndMode=Last  ColEndIndex=1
  Extract Sync1 : dspmtrx3/Submatrix  RowSpan=One row  RowStartMode=First  RowStartIndex=1  RowEndMode=Index  RowEndIndex=8  ColSpan=All columns  ColStartMode=First  ColStartIndex=1  ColEndMode=Last  ColEndIndex=1
  Extract Sync2 : dspmtrx3/Submatrix  RowSpan=One row  RowStartMode=Index  RowStartIndex=188+1  RowEndMode=Index  RowEndIndex=8  ColSpan=All columns  ColStartMode=First  ColStartIndex=1  ColEndMode=Last  ColEndIndex=1
  Extract Sync3 : dspmtrx3/Submatrix  RowSpan=One row  RowStartMode=Index  RowStartIndex=2*188+1  RowEndMode=Index  RowEndIndex=8  ColSpan=All columns  ColStartMode=First  ColStartIndex=1  ColEndMode=Last  ColEndIndex=1
  Extract Sync4 : dspmtrx3/Submatrix  RowSpan=One row  RowStartMode=Index  RowStartIndex=3*188+1  RowEndMode=Index  RowEndIndex=8  ColSpan=All columns  ColStartMode=First  ColStartIndex=1  ColEndMode=Last  ColEndIndex=1
  Extract Sync5 : dspmtrx3/Submatrix  RowSpan=One row  RowStartMode=Index  RowStartIndex=4*188+1  RowEndMode=Index  RowEndIndex=8  ColSpan=All columns  ColStartMode=First  ColStartIndex=1  ColEndMode=Last  ColEndIndex=1
  Extract Sync6 : dspmtrx3/Submatrix  RowSpan=One row  RowStartMode=Index  RowStartIndex=5*188+1  RowEndMode=Index  RowEndIndex=8  ColSpan=All columns  ColStartMode=First  ColStartIndex=1  ColEndMode=Last  ColEndIndex=1
  Extract Sync7 : dspmtrx3/Submatrix  RowSpan=One row  RowStartMode=Index  RowStartIndex=6*188+1  RowEndMode=Index  RowEndIndex=8  ColSpan=All columns  ColStartMode=First  ColStartIndex=1  ColEndMode=Last  ColEndIndex=1
  Extract Sync8 : dspmtrx3/Submatrix  RowSpan=One row  RowStartMode=Index  RowStartIndex=7*188+1  RowEndMode=Index  RowEndIndex=8  ColSpan=All columns  ColStartMode=First  ColStartIndex=1  ColEndMode=Last  ColEndIndex=1
  Matrix Concatenate : Concatenate  NumInputs=16  Mode=Multidimensional array
  Sync1 Inversion : simulink/Logic and Bit Operations/Bitwise Operator  logicop=NOT  UseBitMask=off  BitMask=bin2dec('11011001')  BitMaskRealWorld=Stored Integer
  XOR{,1..7} (8 alike) : simulink/Logic and Bit Operations/Bitwise Operator  logicop=XOR  UseBitMask=off  NumInputPorts=2  BitMask=bin2dec('11011001')  BitMaskRealWorld=Stored Integer
  Out1 : Outport
  wires:
  [SuperFrame] -> Extract Pkt2 Data/1, Extract Pkt3 Data/1, Extract Pkt4 Data/1, Extract Pkt5 Data/1, Extract Pkt6 Data/1, Extract Pkt8 Data/1, Extract Sync8/1, Extract Pkt7 Data/1, Extract Sync7/1, Extract Sync6/1, Extract Sync5/1, Extract Sync4/1, Extract Sync3/1, Extract Sync2/1, Extract Pkt1 Data Bytes 2 to 188/1, Extract Sync1/1
  Extract Sync1/1 -> Sync1 Inversion/1
  Extract Pkt1 Data Bytes 2 to 188/1 -> XOR/2
  [PNSeq_1_187] -> XOR/1
  Sync1 Inversion/1 -> Matrix Concatenate/1
  XOR/1 -> Matrix Concatenate/2
  Extract Sync2/1 -> Matrix Concatenate/3
  Extract Sync3/1 -> Matrix Concatenate/5
  Extract Sync4/1 -> Matrix Concatenate/7
  Extract Sync5/1 -> Matrix Concatenate/9
  Extract Sync6/1 -> Matrix Concatenate/11
  Extract Sync7/1 -> Matrix Concatenate/13
  Extract Sync8/1 -> Matrix Concatenate/15
  XOR1/1 -> Matrix Concatenate/4
  XOR2/1 -> Matrix Concatenate/6
  XOR3/1 -> Matrix Concatenate/8
  XOR4/1 -> Matrix Concatenate/10
  XOR5/1 -> Matrix Concatenate/12
  XOR6/1 -> Matrix Concatenate/14
  XOR7/1 -> Matrix Concatenate/16
  [PNSeq_189_375] -> XOR1/1
  [PNSeq_377_563] -> XOR2/1
  [PNSeq_565_751] -> XOR3/1
  [PNSeq_753_939] -> XOR4/1
  [PNSeq_941_1127] -> XOR5/1
  [PNSeq_1129_1315] -> XOR6/1
  [PNSeq_1317_1503] -> XOR7/1
  Extract Pkt2 Data/1 -> XOR1/2
  Extract Pkt3 Data/1 -> XOR2/2
  Extract Pkt4 Data/1 -> XOR3/2
  Extract Pkt5 Data/1 -> XOR4/2
  Extract Pkt6 Data/1 -> XOR5/2
  Extract Pkt7 Data/1 -> XOR6/2
  Extract Pkt8 Data/1 -> XOR7/2
  Matrix Concatenate/1 -> Out1/1
  PRBS1/1 -> [PNSeq_1_187]
  PRBS2/1 -> [PNSeq_189_375]
  PRBS3/1 -> [PNSeq_377_563]
  PRBS4/1 -> [PNSeq_565_751]
  PRBS5/1 -> [PNSeq_753_939]
  PRBS6/1 -> [PNSeq_941_1127]
  PRBS7/1 -> [PNSeq_1129_1315]
  PRBS8/1 -> [PNSeq_1317_1503]
  Data/1 -> [SuperFrame]
